simulink model "sin"  (R2023b)
settings: Solver=VariableStepAuto  StartTime=0.0  StopTime=10.0  RelTol=1e-3
settings Model: Creator=1234  LastModifiedBy=1234

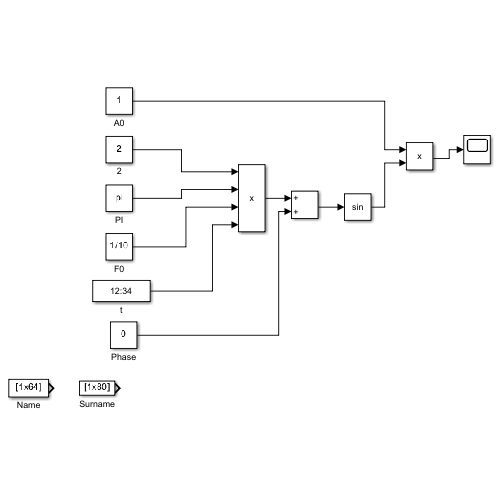
[thumbnail: Simulink's stored preview of the top-level diagram]
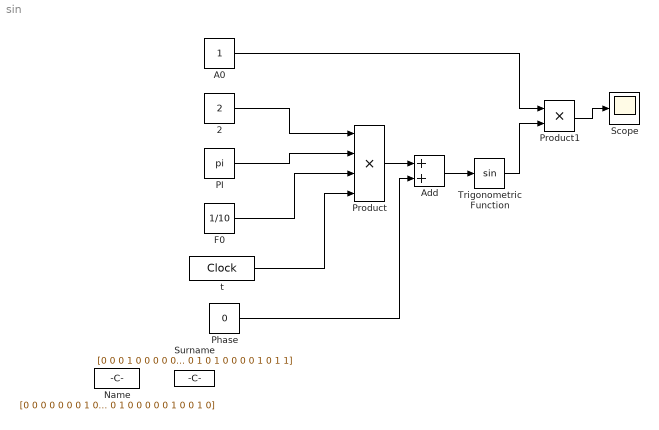
== system sin ==
  2 : Constant  Value=2
  A0 : Constant
  Add : Sum
  F0 : Constant  Value=1/10
  Name : Constant  Value=[0 0 0 0 0 0 0 1 0 0 0 0 1 1 0 0 0 0 0 0 0 1 0 1 0 0 0 1 1 0 0 0 0 0 0 0 0 0 0 1 0 0 0 0 1 1 1 0 0 0 0 0 0 1 0 0 0 0 0 1 0 0 1 0]
  PI : Constant  Value=pi
  Phase : Constant  Value=0
  Product : Product  Inputs=4
  Product1 : Product
  Scope : Scope
  Surname : Constant  Value=[0 0 0 1 0 0 0 0 0 0 0 0 1 1 1 1 0 0 0 0 0 1 1 1 0 0 0 1 0 0 1 0 0 0 0 0 0 1 0 1 0 0 0 0 0 0 1 0 0 0 0 0 1 1 1 0 0 0 0 1 1 0 0 1 0 0 0 1 0 1 0 1 0 0 0 0 1 0 1 1]
  Trigonometric Function : Trigonometry
  t : DigitalClock  SampleTime=1/20
  wires:
  2/1 -> Product/1
  PI/1 -> Product/2
  F0/1 -> Product/3
  t/1 -> Product/4
  Phase/1 -> Add/2
  Product/1 -> Add/1
  Add/1 -> Trigonometric Function/1
  Trigonometric Function/1 -> Product1/2
  A0/1 -> Product1/1
  Product1/1 -> Scope/1
